simulink model "mv_usv_2dof_quad_drag_ssmethod_tcurve"  (R2015b)
settings: Solver=VariableStepAuto  StartTime=0.0  StopTime=200  RelTol=1e-3
values from neighbouring files (symbols this model uses):
  breakpoints1 = data(end:-1:1,1)'    [Experimental_Impl.m]    (also in Experimental_Impl_wPlot.m; FEB02_LAKE_TEST.m; FEB14_LAKE_TEST.m; FEB28_LAKE_TEST.m)
  table_data = data(end:-1:1,2)'    [Experimental_Impl.m]    (also in Experimental_Impl_wPlot.m; FEB02_LAKE_TEST.m; FEB14_LAKE_TEST.m; FEB28_LAKE_TEST.m)
settings Model: Creator=bsb  LastModifiedBy=aschnieders22
settings ConfigComp: CovModelRefEnable=Off
settings ConfigurationSet: Description=Simscape Multibody

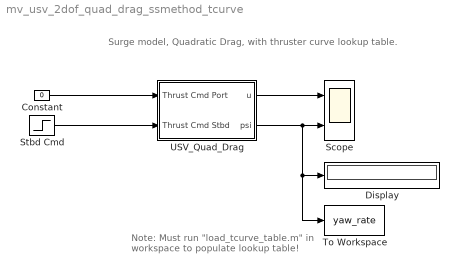
== system mv_usv_2dof_quad_drag_ssmethod_tcurve ==
  note: Note: Must run "load_tcurve_table.m" in workspace to populate lookup table!
  note: Surge model, Quadratic Drag, with thruster curve lookup table.
  Constant : Constant  Value=0
  Display : Display
  Scope : Scope  NumInputPorts=2
  Stbd Cmd : Step  SampleTime=0
  To Workspace : ToWorkspace  VariableName=yaw_rate  SaveFormat=Timeseries  SampleTime=-1
  USV_Quad_Drag : Subsystem
  wires:
  USV_Quad_Drag/1(u) -> Scope/1
  USV_Quad_Drag/2(psi) -> Display/1, To Workspace/1, Scope/2
  Constant/1 -> USV_Quad_Drag/1(Thrust Cmd Port)
  Stbd Cmd/1 -> USV_Quad_Drag/2(Thrust Cmd Stbd)

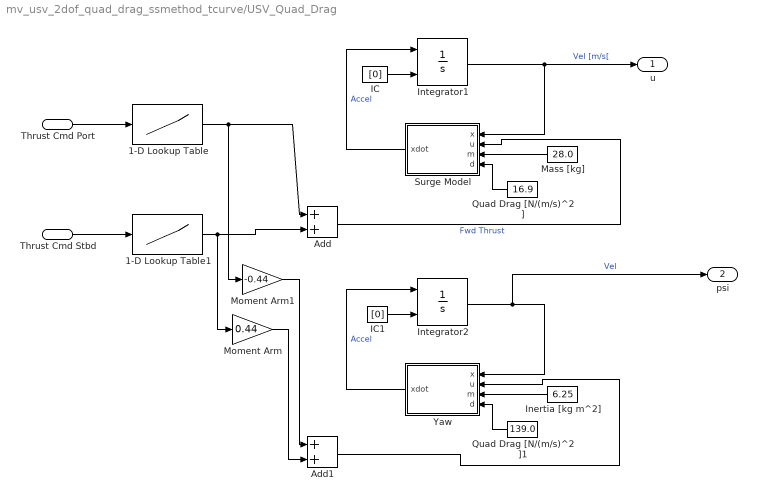
== system mv_usv_2dof_quad_drag_ssmethod_tcurve/USV_Quad_Drag ==
  Thrust Cmd Port : Inport
  Thrust Cmd Stbd : Inport  Port=2
  1-D Lookup Table : Lookup_n-D  NumberOfTableDimensions=1  BreakpointsForDimension1=breakpoints1  Table=table_data  ExtrapMethod=Clip  UseLastTableValue=on  InternalRulePriority=Speed  RndMeth=Simplest  InputSameDT=on
  1-D Lookup Table1 : Lookup_n-D  NumberOfTableDimensions=1  BreakpointsForDimension1=breakpoints1  Table=table_data  ExtrapMethod=Clip  UseLastTableValue=on  InternalRulePriority=Speed  RndMeth=Simplest  InputSameDT=on
  Add : Sum
  Add1 : Sum
  IC : Constant  Value=[0]
  IC1 : Constant  Value=[0]
  Inertia [kg m^2] : Constant  Value=6.25
  Integrator1 : Integrator  InitialConditionSource=external
  Integrator2 : Integrator  InitialConditionSource=external
  Mass [kg] : Constant  Value=28.0
  Moment Arm : Gain  Gain=0.44
  Moment Arm1 : Gain  Gain=-0.44
  Quad Drag [N/(m/s)^2] : Constant  Value=16.9
  Quad Drag [N/(m/s)^2]1 : Constant  Value=139.0
  Surge Model : MATLAB Function  TreatAsAtomicUnit=on
  Yaw : MATLAB Function  TreatAsAtomicUnit=on
  u : Outport
  psi : Outport  Port=2
  wires:
  IC/1 -> Integrator1/2
  Surge Model/1(xdot) -> Integrator1/1  "Accel"
  Integrator1/1 -> u/1, Surge Model/1(x)  "Vel [m/s["
  Add/1 -> Surge Model/2(u)  "Fwd Thrust"
  1-D Lookup Table/1 -> Moment Arm1/1, Add/1
  Thrust Cmd Port/1 -> 1-D Lookup Table/1
  Mass [kg]/1 -> Surge Model/3(m)
  Quad Drag [N/(m/s)^2]/1 -> Surge Model/4(d)
  1-D Lookup Table1/1 -> Moment Arm/1, Add/2
  Thrust Cmd Stbd/1 -> 1-D Lookup Table1/1
  IC1/1 -> Integrator2/2
  Yaw/1(xdot) -> Integrator2/1  "Accel"
  Integrator2/1 -> psi/1, Yaw/1(x)  "Vel"
  Inertia [kg m^2]/1 -> Yaw/3(m)
  Quad Drag [N/(m/s)^2]1/1 -> Yaw/4(d)
  Moment Arm1/1 -> Add1/1
  Moment Arm/1 -> Add1/2
  Add1/1 -> Yaw/2(u)

== matlab function mv_usv_2dof_quad_drag_ssmethod_tcurve/USV_Quad_Drag/Yaw ==
  data: x input; u input; xdot output; m input; d input
function xdot = fcn(x,u,m,d)
%#codegen

% x - state of the system.  surge velocity.
% u - input. thrust force
% Model parameters
m = m; %28.0;   % Mass [kg]
d = d; %16.9;  % Quadratic drag coefficient [N/(m/s)^2]

xdot = 1/m*(-d*abs(x)*x+u);

== matlab function mv_usv_2dof_quad_drag_ssmethod_tcurve/USV_Quad_Drag/Surge Model ==
  data: x input; u input; xdot output; m input; d input
function xdot = fcn(x,u,m,d)
%#codegen

% x - state of the system.  surge velocity.
% u - input. thrust force
% Model parameters
m = m; %28.0;   % Mass [kg]
d = d; %16.9;  % Quadratic drag coefficient [N/(m/s)^2]

xdot = 1/m*(-d*abs(x)*x+u);
